simulink model "untitled"  (R2023a)
settings: Solver=VariableStepAuto  StartTime=0.0  StopTime=1  MaxStep=1e-5  RelTol=1e-3
values from neighbouring files (symbols this model uses):
  A = [0 1; 0 -p]    [realimentador.m]
  B = [0; ke]    [realimentador.m]
  C = [1, 0]    [realimentador.m]
  ke = 5.6318e3    (= 5631.8)    [realimentador.m]
  Ki = acker(Aamp, Bamp, [-0.5*p, -0.5*p, -0.7*p])    [realimentador.m]
  L = acker(A', C', [-1.2*p, -1.2*p])'    [realimentador.m]
  p = 50.8042    [realimentador.m]
settings Model: Creator=erwinplanck  LastModifiedBy=erwinplanck

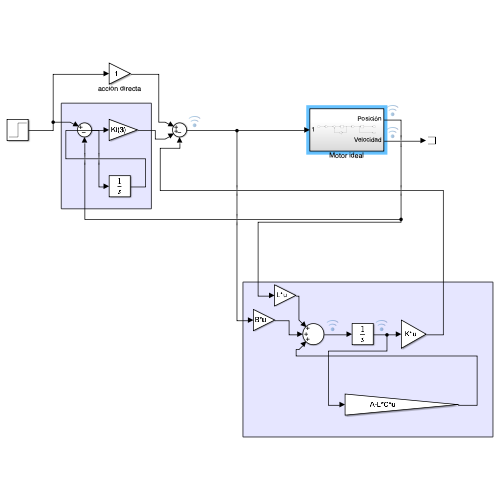
[thumbnail: Simulink's stored preview of the top-level diagram]
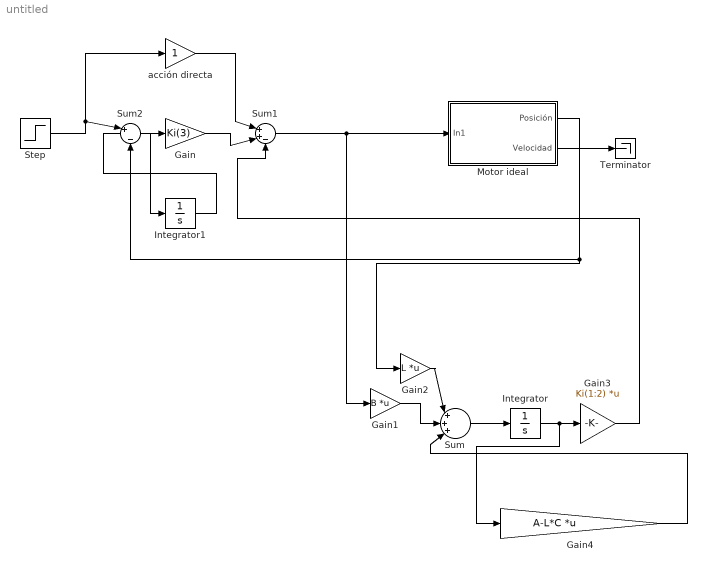
== system untitled ==
  Gain : Gain  Gain=Ki(3)
  Gain1 : Gain  Gain=B  Multiplication=Matrix(K*u)
  Gain2 : Gain  Gain=L  Multiplication=Matrix(K*u)
  Gain3 : Gain  Gain=Ki(1:2)  Multiplication=Matrix(K*u)
  Gain4 : Gain  Gain=A-L*C  Multiplication=Matrix(K*u)
  Integrator : Integrator
  Integrator1 : Integrator
  Motor ideal : Subsystem
  Step : Step  Time=0  After=0  SampleTime=0
  Sum : Sum  Inputs=|+++|
  Sum1 : Sum  Inputs=|++-
  Sum2 : Sum  Inputs=|+|-
  Terminator : Terminator
  acción directa : Gain
  wires:
  Sum1/1 -> Motor ideal/1(In1), Gain1/1
  Motor ideal/1(Posición) -> Sum2/2, Gain2/1
  Motor ideal/2(Velocidad) -> Terminator/1
  Step/1 -> Sum2/1, acción directa/1
  acción directa/1 -> Sum1/1
  Gain2/1 -> Sum/1
  Gain1/1 -> Sum/2
  Sum/1 -> Integrator/1
  Integrator/1 -> Gain4/1, Gain3/1
  Gain3/1 -> Sum1/3
  Gain4/1 -> Sum/3
  Sum2/1 -> Integrator1/1
  Integrator1/1 -> Gain/1
  Gain/1 -> Sum1/2

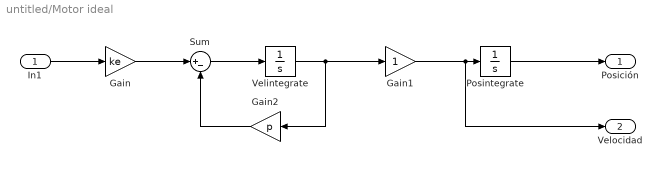
== system untitled/Motor ideal ==
  In1 : Inport
  Gain : Gain  Gain=ke
  Gain1 : Gain
  Gain2 : Gain  Gain=p
  Posintegrate : Integrator
  Sum : Sum  Inputs=|+-
  Velintegrate : Integrator  InitialCondition=4
  Posición : Outport
  Velocidad : Outport  Port=2
  wires:
  Sum/1 -> Velintegrate/1
  Gain2/1 -> Sum/2
  Gain1/1 -> Velocidad/1, Posintegrate/1
  Posintegrate/1 -> Posición/1
  In1/1 -> Gain/1
  Velintegrate/1 -> Gain2/1, Gain1/1
  Gain/1 -> Sum/1
